simulink model "phm_aug5_powertrain"  (R2019a)
settings: Solver=VariableStepAuto  StartTime=0.0  StopTime=1000  FixedStep=.01  RelTol=1e-3
InitFcn:
  | addpath fcns;
  | load batteryParams;
  | load motorParams;
  | load ukfBatteryParams;
  | load ukfMotorParams;
libraries: simulink x6, dspstat3 x1
settings Model: Creator=tdarrah  LastModifiedBy=tdarrah
settings SolverCC: ShapePreserveControl=EnableAll  AlgebraicLoopSolver=LineSearch
settings DebuggingCC: ArithmeticOperatorsInVariantConditions=warning

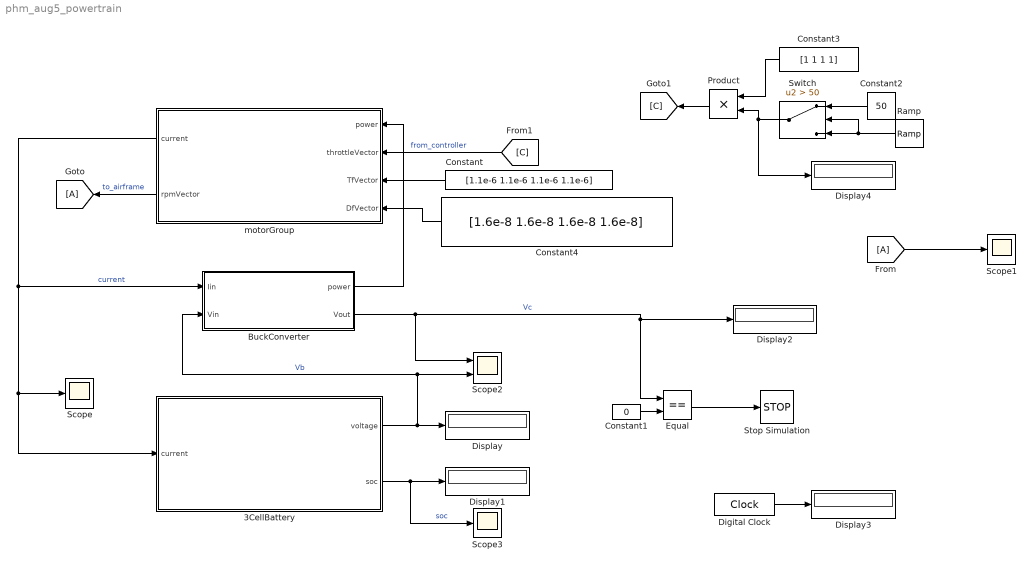
== system phm_aug5_powertrain ==
  3CellBattery : Subsystem
  BuckConverter : Subsystem
  Constant : Constant  Value=[1.1e-6 1.1e-6 1.1e-6 1.1e-6]
  Constant1 : Constant  Value=0
  Constant2 : Constant  Value=50
  Constant3 : Constant  Value=[1 1 1 1]
  Constant4 : Constant  Value=[1.6e-8 1.6e-8 1.6e-8 1.6e-8]
  Digital Clock : DigitalClock
      mask Display: disp('Sim Time');
  Display{,1..4} (5 alike) : Display
  Equal : RelationalOperator  Operator===  OutDataTypeStr=boolean  RndMeth=Simplest
  Product : Product
  Ramp : simulink/Sources/Ramp  slope=1  start=0  InitialOutput=0
  Scope : Scope
  Scope1 : Scope
  Scope2 : Scope  NumInputPorts=2
  Scope3 : Scope
  Stop Simulation : Stop
  Switch : Switch  Criteria=u2 > Threshold  Threshold=50
  motorGroup : Subsystem
  wires:
  3CellBattery/1(voltage) -> BuckConverter/2(Vin), Scope2/2, Display/1  "Vb"
  3CellBattery/2(soc) -> Display1/1, Scope3/1  "soc"
  motorGroup/1(current) -> BuckConverter/1(Iin), 3CellBattery/1(current), Scope/1  "current"
  BuckConverter/1(power) -> motorGroup/1(power)
  BuckConverter/2(Vout) -> Equal/1, Display2/1, Scope2/1  "Vc"
  Product/1 -> [C]
  Constant/1 -> motorGroup/3(TfVector)
  motorGroup/2(rpmVector) -> [A]  "to_airframe"
  Constant1/1 -> Equal/2
  Equal/1 -> Stop Simulation/1
  Digital Clock/1 -> Display3/1
  Ramp/1 -> Switch/2, Switch/3
  Constant2/1 -> Switch/1
  Constant3/1 -> Product/1
  Switch/1 -> Display4/1, Product/2
  [C] -> motorGroup/2(throttleVector)  "from_controller"
  [A] -> Scope1/1
  Constant4/1 -> motorGroup/4(DfVector)

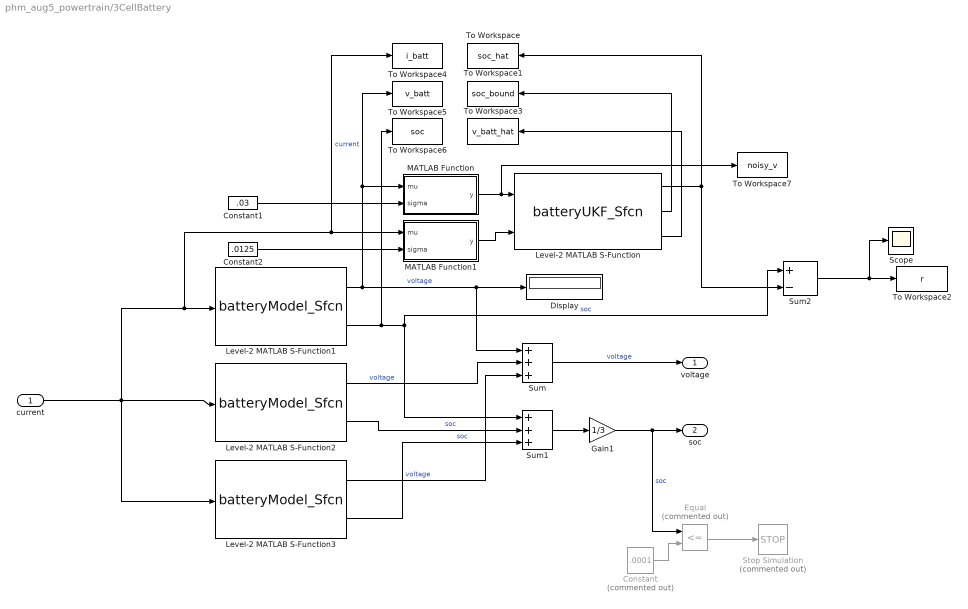
== system phm_aug5_powertrain/3CellBattery ==
  current : Inport
  Constant : Constant  Commented=on  Value=.0001
  Constant1 : Constant  Value=.03
  Constant2 : Constant  Value=.0125
  Display : Display
  Equal : RelationalOperator  Commented=on  Operator=<=  OutDataTypeStr=boolean  RndMeth=Simplest
  Gain1 : Gain  Gain=1/3
  Level-2 MATLAB S-Function : M-S-Function  FunctionName=batteryUKF_Sfcn  Parameters=batteryParams, batteryParams.dt, ukfBatteryParams
      mask Display:
      | port_label('input', 1, 'voltage');
      | port_label('input', 2, 'current');
      | port_label('output', 1, 'soc_hat');
      | port_label('output', 2, 'soc_bound');
      | port_label('output', 3, 'voltage_hat');
      | 
      | disp("UKF");
  Level-2 MATLAB S-Function1 : M-S-Function  FunctionName=batteryModel_Sfcn  Parameters=batteryParams, batteryParams.dt
      mask Display:
      | port_label('input', 1, 'current');
      | port_label('output', 1, 'voltage');
      | port_label('output', 2, 'soc');
      | 
      | disp("Battery Cell");
  Level-2 MATLAB S-Function2 : M-S-Function  FunctionName=batteryModel_Sfcn  Parameters=batteryParams, batteryParams.dt
      mask Display:
      | port_label('input', 1, 'current');
      | port_label('output', 1, 'voltage');
      | port_label('output', 2, 'soc');
  Level-2 MATLAB S-Function3 : M-S-Function  FunctionName=batteryModel_Sfcn  Parameters=batteryParams, batteryParams.dt
      mask Display:
      | port_label('input', 1, 'current');
      | port_label('output', 1, 'voltage');
      | port_label('output', 2, 'soc');
  MATLAB Function : MATLAB Function  TreatAsAtomicUnit=on
  MATLAB Function1 : MATLAB Function  TreatAsAtomicUnit=on
  Scope : Scope
  Stop Simulation : Stop  Commented=on
  Sum : Sum  Inputs=+++
  Sum1 : Sum  Inputs=+++
  Sum2 : Sum  Inputs=+-
  To Workspace : ToWorkspace  VariableName=soc_hat  SaveFormat=Timeseries  SampleTime=-1
  To Workspace1 : ToWorkspace  VariableName=soc_bound  SaveFormat=Timeseries  SampleTime=-1
  To Workspace2 : ToWorkspace  VariableName=r  SaveFormat=Timeseries  SampleTime=-1
  To Workspace3 : ToWorkspace  VariableName=v_batt_hat  SaveFormat=Timeseries  SampleTime=-1
  To Workspace4 : ToWorkspace  VariableName=i_batt  SaveFormat=Timeseries  SampleTime=-1
  To Workspace5 : ToWorkspace  VariableName=v_batt  SaveFormat=Timeseries  SampleTime=-1
  To Workspace6 : ToWorkspace  VariableName=soc  SaveFormat=Timeseries  SampleTime=-1
  To Workspace7 : ToWorkspace  VariableName=noisy_v  SaveFormat=Timeseries  SampleTime=-1
  voltage : Outport
  soc : Outport  Port=2
  wires:
  Level-2 MATLAB S-Function2/1 -> Sum/2  "voltage"
  Level-2 MATLAB S-Function1/1 -> Display/1, Sum/1, MATLAB Function/1(mu), To Workspace5/1  "voltage"
  Level-2 MATLAB S-Function2/2 -> Sum1/2  "soc"
  Sum1/1 -> Gain1/1
  Gain1/1 -> Equal/1, soc/1  "soc"
  Level-2 MATLAB S-Function1/2 -> To Workspace6/1, Sum2/1, Sum1/1  "soc"
  Level-2 MATLAB S-Function3/2 -> Sum1/3  "soc"
  current/1 -> Level-2 MATLAB S-Function3/1, MATLAB Function1/1(mu), To Workspace4/1, Level-2 MATLAB S-Function1/1, Level-2 MATLAB S-Function2/1  "current"
  Level-2 MATLAB S-Function3/1 -> Sum/3  "voltage"
  Sum/1 -> voltage/1  "voltage"
  Constant/1 -> Equal/2
  Equal/1 -> Stop Simulation/1
  Level-2 MATLAB S-Function/1 -> Sum2/2, To Workspace/1
  Level-2 MATLAB S-Function/2 -> To Workspace1/1
  Sum2/1 -> Scope/1, To Workspace2/1
  Level-2 MATLAB S-Function/3 -> To Workspace3/1
  Constant1/1 -> MATLAB Function/2(sigma)
  MATLAB Function/1(y) -> To Workspace7/1, Level-2 MATLAB S-Function/1
  MATLAB Function1/1(y) -> Level-2 MATLAB S-Function/2
  Constant2/1 -> MATLAB Function1/2(sigma)

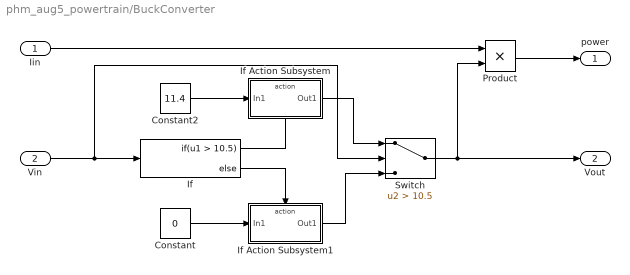
== system phm_aug5_powertrain/BuckConverter ==
  Iin : Inport
  Vin : Inport  Port=2
  Constant : Constant  Value=0
  Constant2 : Constant  Value=11.4
  If : If  IfExpression=u1 > 10.5
  If Action Subsystem : Subsystem  TreatAsAtomicUnit=on
  If Action Subsystem1 : Subsystem  TreatAsAtomicUnit=on
  Product : Product
  Switch : Switch  Criteria=u2 > Threshold  Threshold=10.5
  power : Outport
  Vout : Outport  Port=2
  wires:
  Product/1 -> power/1
  Iin/1 -> Product/1
  If/1 -> If Action Subsystem/Action
  If/2 -> If Action Subsystem1/Action
  Constant/1 -> If Action Subsystem1/1(In1)
  If Action Subsystem/1(Out1) -> Switch/1
  If Action Subsystem1/1(Out1) -> Switch/3
  Constant2/1 -> If Action Subsystem/1(In1)
  Vin/1 -> Switch/2, If/1
  Switch/1 -> Product/2, Vout/1

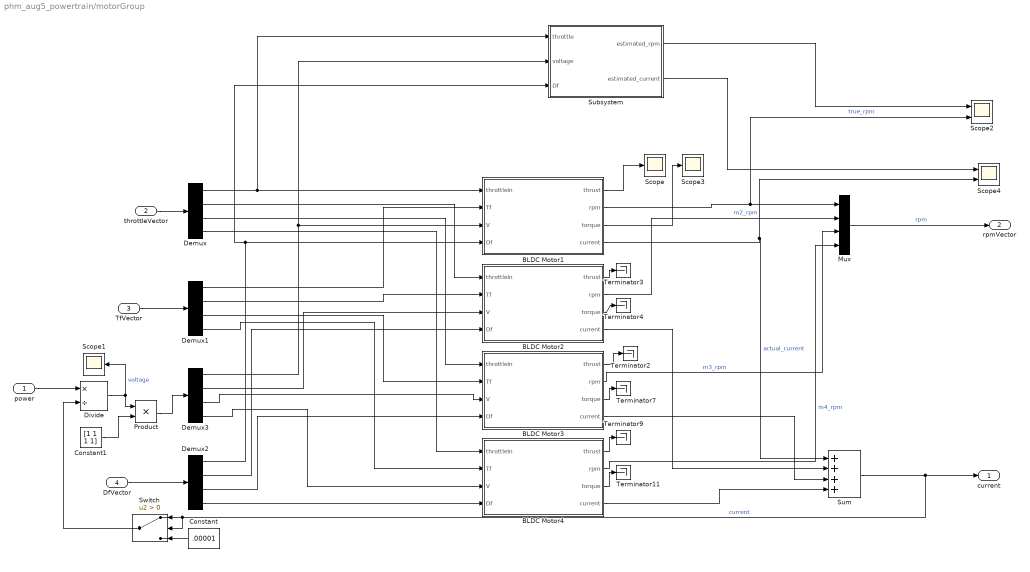
== system phm_aug5_powertrain/motorGroup ==
  power : Inport
  throttleVector : Inport  Port=2  PortDimensions=4
  TfVector : Inport  Port=3  PortDimensions=4
  DfVector : Inport  Port=4
  BLDC Motor1 : Subsystem
  BLDC Motor2 : Subsystem
  BLDC Motor3 : Subsystem
  BLDC Motor4 : Subsystem
  Constant : Constant  Value=.00001
  Constant1 : Constant  Value=[1 1 1 1]
  Demux{,1..3} (4 alike) : Demux
  Divide : Product  Inputs=*/
  Mux : Mux
  Product : Product
  Scope : Scope
  Scope1 : Scope
  Scope2 : Scope  NumInputPorts=2
  Scope3 : Scope
  Scope4 : Scope  NumInputPorts=2
  Subsystem : Subsystem
  Sum : Sum  Inputs=++++
  Switch : Switch  Criteria=u2 > Threshold
  Terminator{2..4,7,9,11} (6 alike) : Terminator
  current : Outport
  rpmVector : Outport  Port=2
  wires:
  Demux1/2 -> BLDC Motor2/2(Tf)
  Demux1/4 -> BLDC Motor4/2(Tf)
  Divide/1 -> Scope1/1, Product/1  "voltage"
  Demux1/1 -> BLDC Motor1/2(Tf)
  Sum/1 -> Switch/2, Switch/1, current/1  "current"
  Demux1/3 -> BLDC Motor3/2(Tf)
  BLDC Motor1/4(current) -> Scope4/2, Sum/1  "actual_current"
  power/1 -> Divide/1
  Demux/4 -> BLDC Motor4/1(throttleIn)
  Demux/3 -> BLDC Motor3/1(throttleIn)
  Demux/2 -> BLDC Motor2/1(throttleIn)
  throttleVector/1 -> Demux/1
  TfVector/1 -> Demux1/1
  BLDC Motor4/4(current) -> Sum/4
  BLDC Motor3/4(current) -> Sum/3
  BLDC Motor2/4(current) -> Sum/2
  BLDC Motor4/2(rpm) -> Mux/4  "m4_rpm"
  BLDC Motor3/2(rpm) -> Mux/3  "m3_rpm"
  BLDC Motor2/2(rpm) -> Mux/2  "m2_rpm"
  BLDC Motor1/2(rpm) -> Scope2/2, Mux/1  "true_rpm"
  Mux/1 -> rpmVector/1  "rpm"
  BLDC Motor1/1(thrust) -> Scope/1
  BLDC Motor4/3(torque) -> Terminator11/1
  BLDC Motor1/3(torque) -> Scope3/1
  BLDC Motor2/3(torque) -> Terminator4/1
  BLDC Motor3/3(torque) -> Terminator7/1
  BLDC Motor4/1(thrust) -> Terminator9/1
  BLDC Motor3/1(thrust) -> Terminator2/1
  BLDC Motor2/1(thrust) -> Terminator3/1
  Switch/1 -> Divide/2
  Constant/1 -> Switch/3
  Demux/1 -> Subsystem/1(throttle), BLDC Motor1/1(throttleIn)
  Subsystem/1(estimated_rpm) -> Scope2/1
  Subsystem/2(estimated_current) -> Scope4/1
  DfVector/1 -> Demux2/1
  Demux2/1 -> BLDC Motor1/4(Df), Subsystem/3(Df)
  Demux2/2 -> BLDC Motor2/4(Df)
  Demux2/3 -> BLDC Motor3/4(Df)
  Demux2/4 -> BLDC Motor4/4(Df)
  Demux3/1 -> Subsystem/2(voltage), BLDC Motor1/3(V)
  Demux3/2 -> BLDC Motor2/3(V)
  Demux3/3 -> BLDC Motor3/3(V)
  Demux3/4 -> BLDC Motor4/3(V)
  Constant1/1 -> Product/2
  Product/1 -> Demux3/1

== system phm_aug5_powertrain/BuckConverter/If Action Subsystem ==
  In1 : Inport
  Action Port : ActionPort  ActionPortLabel=if(u1 > 10.5)
  Out1 : Outport
  wires:
  In1/1 -> Out1/1

== system phm_aug5_powertrain/BuckConverter/If Action Subsystem1 ==
  In1 : Inport
  Action Port : ActionPort  ActionPortLabel=else
  Out1 : Outport
  wires:
  In1/1 -> Out1/1

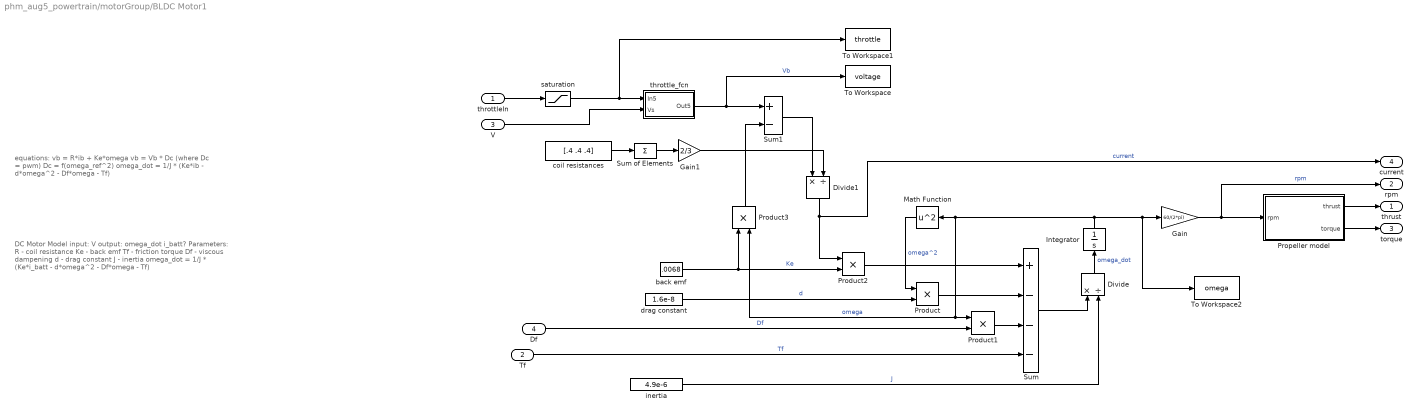
== system phm_aug5_powertrain/motorGroup/BLDC Motor1 ==
  note: DC Motor Model
      |
      | input:
      | V
      |
      | output:
      | omega_dot
      | i_batt?
      |
      |
      | Parameters:
      | R   - coil resistance
      | Ke - back emf
      | Tf  - friction torque
      | Df  - viscous dampening
      | d   - drag constant
      | J   - inertia
      |
      | omega_dot = 1/J * (Ke*i_batt - d*omega^2 - Df*omega - Tf)
  note: equations:
      |
      | vb = R*ib + Ke*omega
      | vb = Vb * Dc  (where Dc = pwm)
      | Dc = f(omega_ref^2)
      |
      | omega_dot = 1/J * (Ke*ib - d*omega^2 - Df*omega - Tf)
  throttleIn : Inport
  Tf : Inport  Port=2
  V : Inport  Port=3
  Df : Inport  Port=4
  Divide : Product  Inputs=*/
  Divide1 : Product  Inputs=*/
  Gain : Gain  Gain=60/(2*pi)
  Gain1 : Gain  Gain=2/3
  Integrator : Integrator
  Math Function : Math  Operator=square  SaturateOnIntegerOverflow=on
  Product{,1..3} (4 alike) : Product
  "Propeller model " : MATLAB Function  TreatAsAtomicUnit=on
  Sum : Sum  Inputs=+---
  Sum of Elements : Sum  Inputs=+
  Sum1 : Sum  Inputs=+-
  To Workspace : ToWorkspace  VariableName=voltage  SaveFormat=Timeseries  SampleTime=-1
  To Workspace1 : ToWorkspace  VariableName=throttle  SaveFormat=Timeseries  SampleTime=-1
  To Workspace2 : ToWorkspace  VariableName=omega  SaveFormat=Timeseries  SampleTime=-1
  back emf : Constant  Value=.0068
  coil resistances : Constant  Value=[.4 .4 .4]
  drag constant : Constant  Value=1.6e-8
  inertia : Constant  Value=4.9e-6
  saturation : Saturate  UpperLimit=100  LowerLimit=0
  throttle_fcn : Subsystem
  thrust : Outport
  rpm : Outport  Port=2
  torque : Outport  Port=3
  current : Outport  Port=4
  wires:
  Divide/1 -> Integrator/1  "omega_dot"
  Integrator/1 -> To Workspace2/1, Gain/1, Math Function/1, Product1/1, Product3/2  "omega"
  Gain/1 -> "Propeller model "/1(rpm), rpm/1  "rpm"
  inertia/1 -> Divide/2  "J"
  drag constant/1 -> Product/2  "d"
  Math Function/1 -> Product/1  "omega^2"
  Df/1 -> Product1/2  "Df"
  Tf/1 -> Sum/4  "Tf"
  back emf/1 -> Product3/1, Product2/2  "Ke"
  Product2/1 -> Sum/1
  Divide1/1 -> current/1, Product2/1  "current"
  V/1 -> throttle_fcn/2(Vs)
  Product3/1 -> Sum1/2
  Sum1/1 -> Divide1/1
  Gain1/1 -> Divide1/2
  "Propeller model "/1(thrust) -> thrust/1
  "Propeller model "/2(torque) -> torque/1
  Product1/1 -> Sum/3
  Product/1 -> Sum/2
  Sum/1 -> Divide/1
  coil resistances/1 -> Sum of Elements/1
  Sum of Elements/1 -> Gain1/1
  throttleIn/1 -> saturation/1
  throttle_fcn/1(Out5) -> To Workspace/1, Sum1/1  "Vb"
  saturation/1 -> To Workspace1/1, throttle_fcn/1(In5)

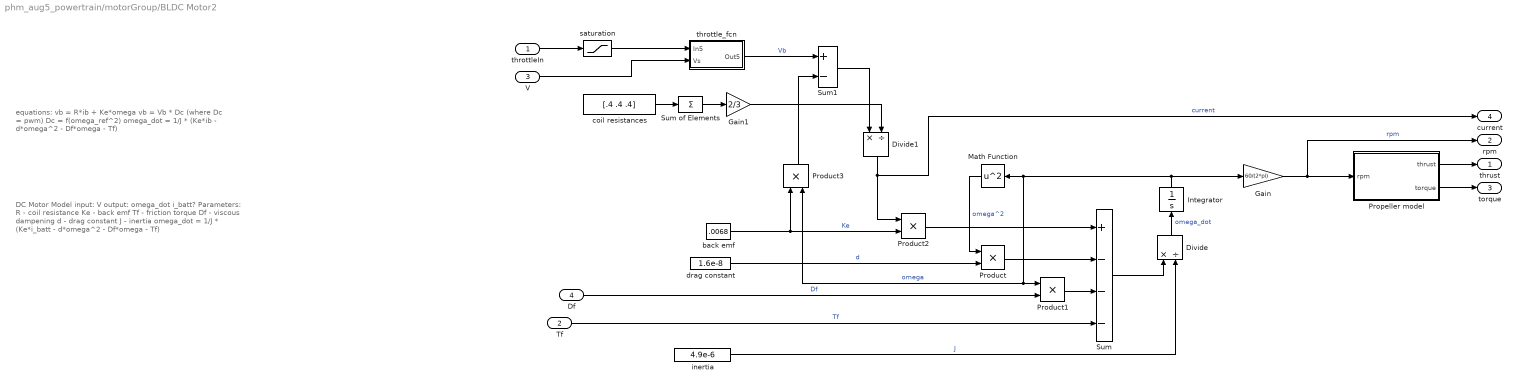
== system phm_aug5_powertrain/motorGroup/BLDC Motor2 ==
  note: DC Motor Model
      |
      | input:
      | V
      |
      | output:
      | omega_dot
      | i_batt?
      |
      |
      | Parameters:
      | R   - coil resistance
      | Ke - back emf
      | Tf  - friction torque
      | Df  - viscous dampening
      | d   - drag constant
      | J   - inertia
      |
      | omega_dot = 1/J * (Ke*i_batt - d*omega^2 - Df*omega - Tf)
  note: equations:
      |
      | vb = R*ib + Ke*omega
      | vb = Vb * Dc  (where Dc = pwm)
      | Dc = f(omega_ref^2)
      |
      | omega_dot = 1/J * (Ke*ib - d*omega^2 - Df*omega - Tf)
  throttleIn : Inport
  Tf : Inport  Port=2
  V : Inport  Port=3
  Df : Inport  Port=4
  Divide : Product  Inputs=*/
  Divide1 : Product  Inputs=*/
  Gain : Gain  Gain=60/(2*pi)
  Gain1 : Gain  Gain=2/3
  Integrator : Integrator
  Math Function : Math  Operator=square  SaturateOnIntegerOverflow=on
  Product{,1..3} (4 alike) : Product
  "Propeller model " : MATLAB Function  TreatAsAtomicUnit=on
  Sum : Sum  Inputs=+---
  Sum of Elements : Sum  Inputs=+
  Sum1 : Sum  Inputs=+-
  back emf : Constant  Value=.0068
  coil resistances : Constant  Value=[.4 .4 .4]
  drag constant : Constant  Value=1.6e-8
  inertia : Constant  Value=4.9e-6
  saturation : Saturate  UpperLimit=100  LowerLimit=0
  throttle_fcn : Subsystem
  thrust : Outport
  rpm : Outport  Port=2
  torque : Outport  Port=3
  current : Outport  Port=4
  wires:
  Divide/1 -> Integrator/1  "omega_dot"
  Integrator/1 -> Gain/1, Math Function/1, Product1/1, Product3/2  "omega"
  Gain/1 -> "Propeller model "/1(rpm), rpm/1  "rpm"
  inertia/1 -> Divide/2  "J"
  drag constant/1 -> Product/2  "d"
  Math Function/1 -> Product/1  "omega^2"
  Df/1 -> Product1/2  "Df"
  Tf/1 -> Sum/4  "Tf"
  back emf/1 -> Product3/1, Product2/2  "Ke"
  Product2/1 -> Sum/1
  Divide1/1 -> current/1, Product2/1  "current"
  V/1 -> throttle_fcn/2(Vs)
  Product3/1 -> Sum1/2
  Sum1/1 -> Divide1/1
  Gain1/1 -> Divide1/2
  "Propeller model "/1(thrust) -> thrust/1
  "Propeller model "/2(torque) -> torque/1
  Product1/1 -> Sum/3
  Product/1 -> Sum/2
  Sum/1 -> Divide/1
  coil resistances/1 -> Sum of Elements/1
  Sum of Elements/1 -> Gain1/1
  throttleIn/1 -> saturation/1
  throttle_fcn/1(Out5) -> Sum1/1  "Vb"
  saturation/1 -> throttle_fcn/1(In5)

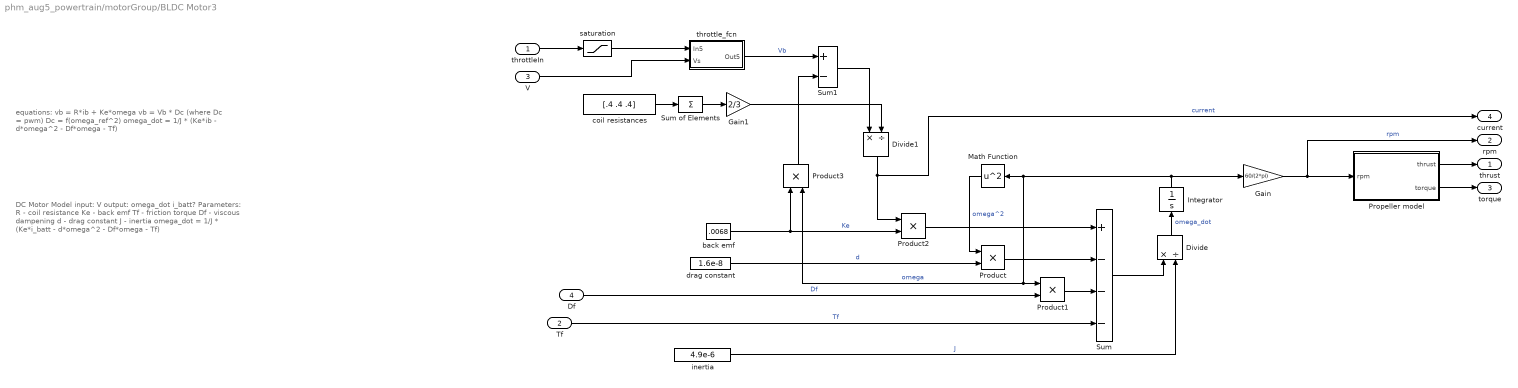
== system phm_aug5_powertrain/motorGroup/BLDC Motor3 ==
  note: DC Motor Model
      |
      | input:
      | V
      |
      | output:
      | omega_dot
      | i_batt?
      |
      |
      | Parameters:
      | R   - coil resistance
      | Ke - back emf
      | Tf  - friction torque
      | Df  - viscous dampening
      | d   - drag constant
      | J   - inertia
      |
      | omega_dot = 1/J * (Ke*i_batt - d*omega^2 - Df*omega - Tf)
  note: equations:
      |
      | vb = R*ib + Ke*omega
      | vb = Vb * Dc  (where Dc = pwm)
      | Dc = f(omega_ref^2)
      |
      | omega_dot = 1/J * (Ke*ib - d*omega^2 - Df*omega - Tf)
  throttleIn : Inport
  Tf : Inport  Port=2
  V : Inport  Port=3
  Df : Inport  Port=4
  Divide : Product  Inputs=*/
  Divide1 : Product  Inputs=*/
  Gain : Gain  Gain=60/(2*pi)
  Gain1 : Gain  Gain=2/3
  Integrator : Integrator
  Math Function : Math  Operator=square  SaturateOnIntegerOverflow=on
  Product{,1..3} (4 alike) : Product
  "Propeller model " : MATLAB Function  TreatAsAtomicUnit=on
  Sum : Sum  Inputs=+---
  Sum of Elements : Sum  Inputs=+
  Sum1 : Sum  Inputs=+-
  back emf : Constant  Value=.0068
  coil resistances : Constant  Value=[.4 .4 .4]
  drag constant : Constant  Value=1.6e-8
  inertia : Constant  Value=4.9e-6
  saturation : Saturate  UpperLimit=100  LowerLimit=0
  throttle_fcn : Subsystem
  thrust : Outport
  rpm : Outport  Port=2
  torque : Outport  Port=3
  current : Outport  Port=4
  wires:
  Divide/1 -> Integrator/1  "omega_dot"
  Integrator/1 -> Gain/1, Math Function/1, Product1/1, Product3/2  "omega"
  Gain/1 -> "Propeller model "/1(rpm), rpm/1  "rpm"
  inertia/1 -> Divide/2  "J"
  drag constant/1 -> Product/2  "d"
  Math Function/1 -> Product/1  "omega^2"
  Df/1 -> Product1/2  "Df"
  Tf/1 -> Sum/4  "Tf"
  back emf/1 -> Product3/1, Product2/2  "Ke"
  Product2/1 -> Sum/1
  Divide1/1 -> current/1, Product2/1  "current"
  V/1 -> throttle_fcn/2(Vs)
  Product3/1 -> Sum1/2
  Sum1/1 -> Divide1/1
  Gain1/1 -> Divide1/2
  "Propeller model "/1(thrust) -> thrust/1
  "Propeller model "/2(torque) -> torque/1
  Product1/1 -> Sum/3
  Product/1 -> Sum/2
  Sum/1 -> Divide/1
  coil resistances/1 -> Sum of Elements/1
  Sum of Elements/1 -> Gain1/1
  throttleIn/1 -> saturation/1
  throttle_fcn/1(Out5) -> Sum1/1  "Vb"
  saturation/1 -> throttle_fcn/1(In5)

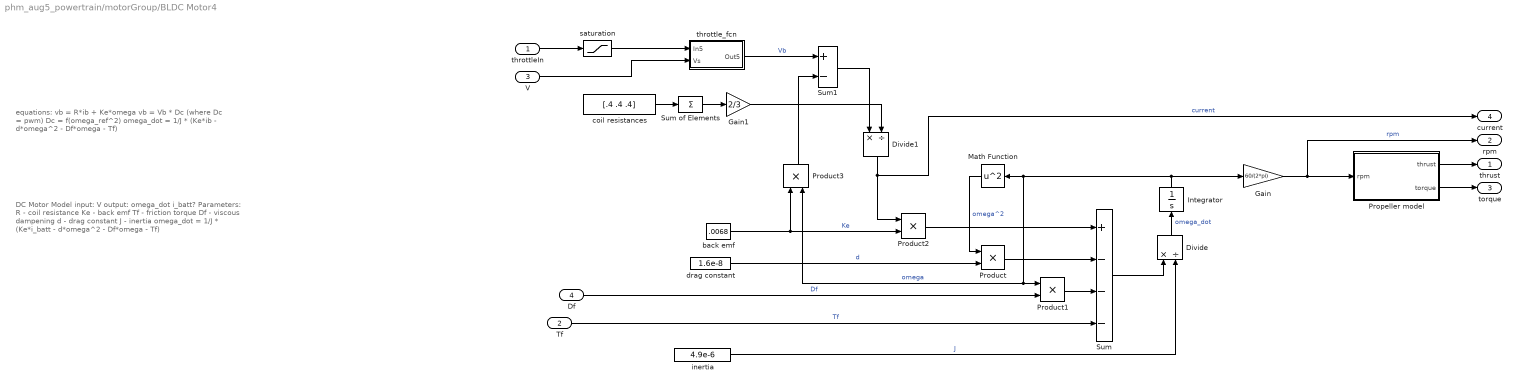
== system phm_aug5_powertrain/motorGroup/BLDC Motor4 ==
  note: DC Motor Model
      |
      | input:
      | V
      |
      | output:
      | omega_dot
      | i_batt?
      |
      |
      | Parameters:
      | R   - coil resistance
      | Ke - back emf
      | Tf  - friction torque
      | Df  - viscous dampening
      | d   - drag constant
      | J   - inertia
      |
      | omega_dot = 1/J * (Ke*i_batt - d*omega^2 - Df*omega - Tf)
  note: equations:
      |
      | vb = R*ib + Ke*omega
      | vb = Vb * Dc  (where Dc = pwm)
      | Dc = f(omega_ref^2)
      |
      | omega_dot = 1/J * (Ke*ib - d*omega^2 - Df*omega - Tf)
  throttleIn : Inport
  Tf : Inport  Port=2
  V : Inport  Port=3
  Df : Inport  Port=4
  Divide : Product  Inputs=*/
  Divide1 : Product  Inputs=*/
  Gain : Gain  Gain=60/(2*pi)
  Gain1 : Gain  Gain=2/3
  Integrator : Integrator
  Math Function : Math  Operator=square  SaturateOnIntegerOverflow=on
  Product{,1..3} (4 alike) : Product
  "Propeller model " : MATLAB Function  TreatAsAtomicUnit=on
  Sum : Sum  Inputs=+---
  Sum of Elements : Sum  Inputs=+
  Sum1 : Sum  Inputs=+-
  back emf : Constant  Value=.0068
  coil resistances : Constant  Value=[.4 .4 .4]
  drag constant : Constant  Value=1.6e-8
  inertia : Constant  Value=4.9e-6
  saturation : Saturate  UpperLimit=100  LowerLimit=0
  throttle_fcn : Subsystem
  thrust : Outport
  rpm : Outport  Port=2
  torque : Outport  Port=3
  current : Outport  Port=4
  wires:
  Divide/1 -> Integrator/1  "omega_dot"
  Integrator/1 -> Gain/1, Math Function/1, Product1/1, Product3/2  "omega"
  Gain/1 -> "Propeller model "/1(rpm), rpm/1  "rpm"
  inertia/1 -> Divide/2  "J"
  drag constant/1 -> Product/2  "d"
  Math Function/1 -> Product/1  "omega^2"
  Df/1 -> Product1/2  "Df"
  Tf/1 -> Sum/4  "Tf"
  back emf/1 -> Product3/1, Product2/2  "Ke"
  Product2/1 -> Sum/1
  Divide1/1 -> current/1, Product2/1  "current"
  V/1 -> throttle_fcn/2(Vs)
  Product3/1 -> Sum1/2
  Sum1/1 -> Divide1/1
  Gain1/1 -> Divide1/2
  "Propeller model "/1(thrust) -> thrust/1
  "Propeller model "/2(torque) -> torque/1
  Product1/1 -> Sum/3
  Product/1 -> Sum/2
  Sum/1 -> Divide/1
  coil resistances/1 -> Sum of Elements/1
  Sum of Elements/1 -> Gain1/1
  throttleIn/1 -> saturation/1
  throttle_fcn/1(Out5) -> Sum1/1  "Vb"
  saturation/1 -> throttle_fcn/1(In5)

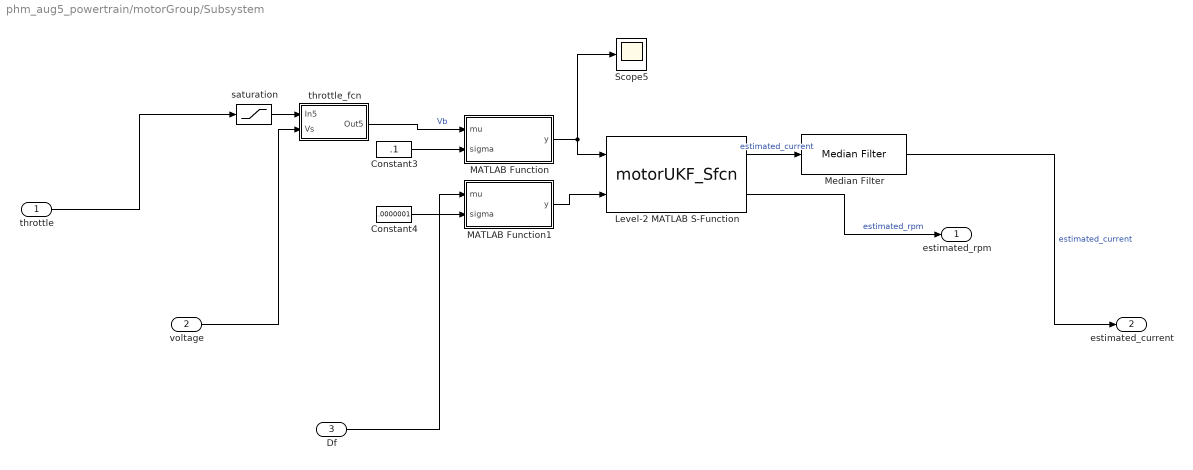
== system phm_aug5_powertrain/motorGroup/Subsystem ==
  throttle : Inport
  voltage : Inport  Port=2
  Df : Inport  Port=3
  Constant3 : Constant  Value=.1
  Constant4 : Constant  Value=.0000001
  Level-2 MATLAB S-Function : M-S-Function  FunctionName=motorUKF_Sfcn  Parameters=motorParams
      mask Display:
      | port_label('input', 1, 'voltage');
      | port_label('input', 2, 'friction');
      | port_label('output', 1, 'current');
      | port_label('output', 2, 'rpm_hat');
      | disp("Motor UKF");
  MATLAB Function : MATLAB Function  TreatAsAtomicUnit=on
  MATLAB Function1 : MATLAB Function  TreatAsAtomicUnit=on
  Median Filter : dspstat3/Median Filter  WindowLength=100  SimulateUsing=Code generation
      settings: SourceProductName=DSP System Toolbox  SourceProductBaseCode=DS
  Scope5 : Scope
  saturation : Saturate  UpperLimit=100  LowerLimit=0
  throttle_fcn : Subsystem
  estimated_rpm : Outport
  estimated_current : Outport  Port=2
  wires:
  Constant4/1 -> MATLAB Function1/2(sigma)
  throttle/1 -> saturation/1
  MATLAB Function/1(y) -> Scope5/1, Level-2 MATLAB S-Function/1
  throttle_fcn/1(Out5) -> MATLAB Function/1(mu)  "Vb"
  Level-2 MATLAB S-Function/2 -> estimated_rpm/1  "estimated_rpm"
  Median Filter/1 -> estimated_current/1  "estimated_current"
  MATLAB Function1/1(y) -> Level-2 MATLAB S-Function/2
  Level-2 MATLAB S-Function/1 -> Median Filter/1  "estimated_current"
  voltage/1 -> throttle_fcn/2(Vs)
  Df/1 -> MATLAB Function1/1(mu)
  saturation/1 -> throttle_fcn/1(In5)
  Constant3/1 -> MATLAB Function/2(sigma)

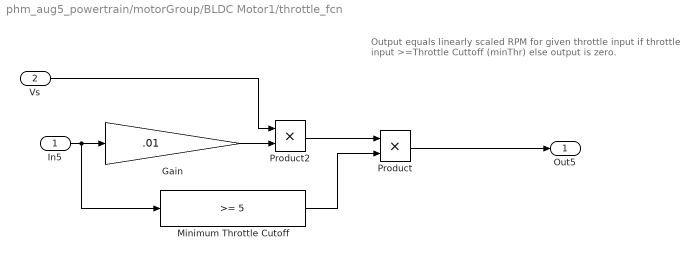
== system phm_aug5_powertrain/motorGroup/BLDC Motor1/throttle_fcn ==
  note: Output equals linearly scaled RPM
      | for given throttle input if throttle input >=Throttle Cuttoff (minThr)
      | else output is zero.
  In5 : Inport
  Vs : Inport  Port=2
  Gain : Gain  Gain=.01
  Minimum Throttle Cutoff : simulink/Logic and Bit Operations/Compare To Constant  relop=>=  const=5  OutDataTypeStr=uint8
  Product : Product
  Product2 : Product  OutDataTypeStr=double
  Out5 : Outport
  wires:
  Minimum Throttle Cutoff/1 -> Product/2
  Product/1 -> Out5/1
  In5/1 -> Gain/1, Minimum Throttle Cutoff/1
  Gain/1 -> Product2/2
  Product2/1 -> Product/1
  Vs/1 -> Product2/1

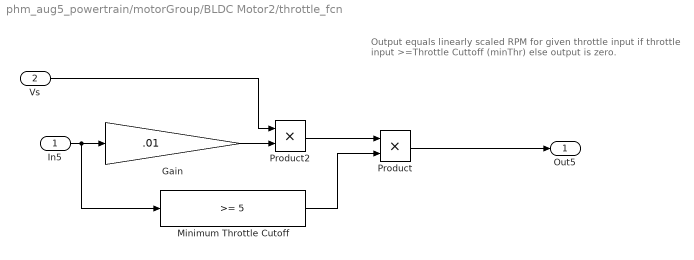
== system phm_aug5_powertrain/motorGroup/BLDC Motor2/throttle_fcn ==
  note: Output equals linearly scaled RPM
      | for given throttle input if throttle input >=Throttle Cuttoff (minThr)
      | else output is zero.
  In5 : Inport
  Vs : Inport  Port=2
  Gain : Gain  Gain=.01
  Minimum Throttle Cutoff : simulink/Logic and Bit Operations/Compare To Constant  relop=>=  const=5  OutDataTypeStr=uint8
  Product : Product
  Product2 : Product  OutDataTypeStr=double
  Out5 : Outport
  wires:
  Minimum Throttle Cutoff/1 -> Product/2
  Product/1 -> Out5/1
  In5/1 -> Gain/1, Minimum Throttle Cutoff/1
  Gain/1 -> Product2/2
  Product2/1 -> Product/1
  Vs/1 -> Product2/1

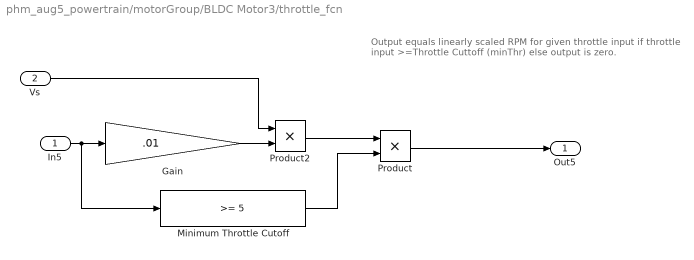
== system phm_aug5_powertrain/motorGroup/BLDC Motor3/throttle_fcn ==
  note: Output equals linearly scaled RPM
      | for given throttle input if throttle input >=Throttle Cuttoff (minThr)
      | else output is zero.
  In5 : Inport
  Vs : Inport  Port=2
  Gain : Gain  Gain=.01
  Minimum Throttle Cutoff : simulink/Logic and Bit Operations/Compare To Constant  relop=>=  const=5  OutDataTypeStr=uint8
  Product : Product
  Product2 : Product  OutDataTypeStr=double
  Out5 : Outport
  wires:
  Minimum Throttle Cutoff/1 -> Product/2
  Product/1 -> Out5/1
  In5/1 -> Gain/1, Minimum Throttle Cutoff/1
  Gain/1 -> Product2/2
  Product2/1 -> Product/1
  Vs/1 -> Product2/1

== system phm_aug5_powertrain/motorGroup/BLDC Motor4/throttle_fcn ==
  note: Output equals linearly scaled RPM
      | for given throttle input if throttle input >=Throttle Cuttoff (minThr)
      | else output is zero.
  In5 : Inport
  Vs : Inport  Port=2
  Gain : Gain  Gain=.01
  Minimum Throttle Cutoff : simulink/Logic and Bit Operations/Compare To Constant  relop=>=  const=5  OutDataTypeStr=uint8
  Product : Product
  Product2 : Product  OutDataTypeStr=double
  Out5 : Outport
  wires:
  Minimum Throttle Cutoff/1 -> Product/2
  Product/1 -> Out5/1
  In5/1 -> Gain/1, Minimum Throttle Cutoff/1
  Gain/1 -> Product2/2
  Product2/1 -> Product/1
  Vs/1 -> Product2/1

== system phm_aug5_powertrain/motorGroup/Subsystem/throttle_fcn ==
  note: Output equals linearly scaled RPM
      | for given throttle input if throttle input >=Throttle Cuttoff (minThr)
      | else output is zero.
  In5 : Inport
  Vs : Inport  Port=2
  Gain : Gain  Gain=.01
  Minimum Throttle Cutoff : simulink/Logic and Bit Operations/Compare To Constant  relop=>=  const=5  OutDataTypeStr=uint8
  Product : Product
  Product2 : Product  OutDataTypeStr=double
  Out5 : Outport
  wires:
  Minimum Throttle Cutoff/1 -> Product/2
  Product/1 -> Out5/1
  In5/1 -> Gain/1, Minimum Throttle Cutoff/1
  Gain/1 -> Product2/2
  Product2/1 -> Product/1
  Vs/1 -> Product2/1

== matlab function phm_aug5_powertrain/3CellBattery/MATLAB Function1 ==
  settings: updateMethod=DISCRETE  sampleTime=.2
  data: mu input; y output; sigma input
function y = addNoise(mu, sigma)

y = normrnd(mu, sigma);

== matlab function phm_aug5_powertrain/3CellBattery/MATLAB Function ==
  settings: updateMethod=DISCRETE  sampleTime=.2
  data: mu input; y output; sigma input
function y = addNoise(mu, sigma)

y = normrnd(mu, sigma);

== matlab function phm_aug5_powertrain/motorGroup/Subsystem/MATLAB Function ==
  settings: updateMethod=DISCRETE  sampleTime=.2
  data: mu input; y output; sigma input
function y = addNoise(mu, sigma)

y = normrnd(mu, sigma);

== matlab function phm_aug5_powertrain/motorGroup/Subsystem/MATLAB Function1 ==
  settings: updateMethod=DISCRETE  sampleTime=.2
  data: mu input; y output; sigma input
function y = addNoise(mu, sigma)

y = normrnd(mu, sigma);

== matlab function phm_aug5_powertrain/motorGroup/BLDC Motor2/Propeller model  ==
  data: thrust output; torque output; rpm input
function [thrust,torque] = fcn(rpm)
% angular_velocity in rpm

%coefficient of thrust, empirically derived
coef_t = 2*(10^-15)*rpm^3 - 4*(10^-11)*rpm^2 + 3*(10^-7)*rpm + .1013;
%thrust = coef_t * density of air * velocity^2 * propeller diameter (m) ^4
thrust = coef_t*1.225*(rpm/60)^2*.2^4;
% empirically derived
torque = 4*(10^-14)*rpm^3 +  8*(10^-12)*rpm^2 + 3*(10^-6)*rpm;
end

== matlab function phm_aug5_powertrain/motorGroup/BLDC Motor3/Propeller model  ==
  data: thrust output; torque output; rpm input
function [thrust,torque] = fcn(rpm)
% angular_velocity in rpm

%coefficient of thrust, empirically derived
coef_t = 2*(10^-15)*rpm^3 - 4*(10^-11)*rpm^2 + 3*(10^-7)*rpm + .1013;
%thrust = coef_t * density of air * velocity^2 * propeller diameter (m) ^4
thrust = coef_t*1.225*(rpm/60)^2*.2^4;
% empirically derived
torque = 4*(10^-14)*rpm^3 +  8*(10^-12)*rpm^2 + 3*(10^-6)*rpm;
end

== matlab function phm_aug5_powertrain/motorGroup/BLDC Motor4/Propeller model  ==
  data: thrust output; torque output; rpm input
function [thrust,torque] = fcn(rpm)
% angular_velocity in rpm

%coefficient of thrust, empirically derived
coef_t = 2*(10^-15)*rpm^3 - 4*(10^-11)*rpm^2 + 3*(10^-7)*rpm + .1013;
%thrust = coef_t * density of air * velocity^2 * propeller diameter (m) ^4
thrust = coef_t*1.225*(rpm/60)^2*.2^4;
% empirically derived
torque = 4*(10^-14)*rpm^3 +  8*(10^-12)*rpm^2 + 3*(10^-6)*rpm;
end

== matlab function phm_aug5_powertrain/motorGroup/BLDC Motor1/Propeller model  ==
  data: thrust output; torque output; rpm input
function [thrust,torque] = fcn(rpm)
% angular_velocity in rpm

%coefficient of thrust, empirically derived
coef_t = 2*(10^-15)*rpm^3 - 4*(10^-11)*rpm^2 + 3*(10^-7)*rpm + .1013;
%thrust = coef_t * density of air * velocity^2 * propeller diameter (m) ^4
thrust = coef_t*1.225*(rpm/60)^2*.2^4;
% empirically derived
torque = 4*(10^-14)*rpm^3 +  8*(10^-12)*rpm^2 + 3*(10^-6)*rpm;
end
